simulink model "ArduCopter"  (R2016a)
settings: Solver=ode8  SolverMode=SingleTasking  StartTime=0.0  StopTime=endtime_selfdefine  FixedStep=0.0025  RelTol=1e-3
InitFcn:
  | %load QuadCopterParameters
values from neighbouring files (symbols this model uses):
  Discretetime_400Hz = 0.0025    [euler_roll_angle_cd.mat]
  flight_mode = 1    [flight_control_run.m]
undefined symbols (not defined in the file or in its folder): Cutoff_frequency_acc_z, D_acc_z, D_vel_x, D_vel_y, DEG_TO_RAD, Discretetime_1Hz, g, I_acc_z, I_vel_x, I_vel_y, Kp_angle, MotorLayout, P_acc_z, P_pos_x, P_pos_y, P_pos_z, P_vel_x, P_vel_y, P_vel_z, thrust_rpyt_down, thrust_rpyt_up
libraries: Lib_AC_AttitudeControl x26, Lib_AP_Math x26, Lib_AP_Motors x5, Lib_AC_PID x4, Lib_AP_AHRS x3, simulink x1
(part 2 of 2)

== system ArduCopter/loop/fast_loop/update_flight_mode/poshold_run/set_throttle_out/update_z_controller/pos_to_rate_z ==
  note: in cm，positive
  _ahrs : Inport
  _pos_target.z : Inport  Port=2
  Bus Selector : BusSelector  OutputSignals=NEDState.Position.zPos,NEDState.Velocity.zVel
  Gain : Gain  Gain=-100
  Gain2 : Gain  Gain=-100
  MATLAB Function1 : Lib_AC_AttitudeControl/MATLAB Function2
  Parameter1 : Constant  Value=P_pos_z  SampleTime=-1
  Parameter2 : Constant  Value=250  SampleTime=-1
  Scope : Scope  NumInputPorts=3
  Subtract : Sum  Inputs=+-
  rate_to_accel_z : Subsystem
  _throttle_in : Outport
  wires:
  _ahrs/1 -> rate_to_accel_z/3(_ahrs), Bus Selector/1
  Bus Selector/1 -> Gain/1  "<zPos>"
  _pos_target.z/1 -> Scope/1, Subtract/1
  Subtract/1 -> MATLAB Function1/1, Scope/3
  Parameter1/1 -> MATLAB Function1/2
  MATLAB Function1/1 -> rate_to_accel_z/1(_vel_target.z)
  Gain2/1 -> rate_to_accel_z/2(_vel_cur.z)
  Bus Selector/2 -> Gain2/1  "<zVel>"
  rate_to_accel_z/1(_throttle_in) -> _throttle_in/1
  Gain/1 -> Scope/2, Subtract/2
  Parameter2/1 -> MATLAB Function1/3

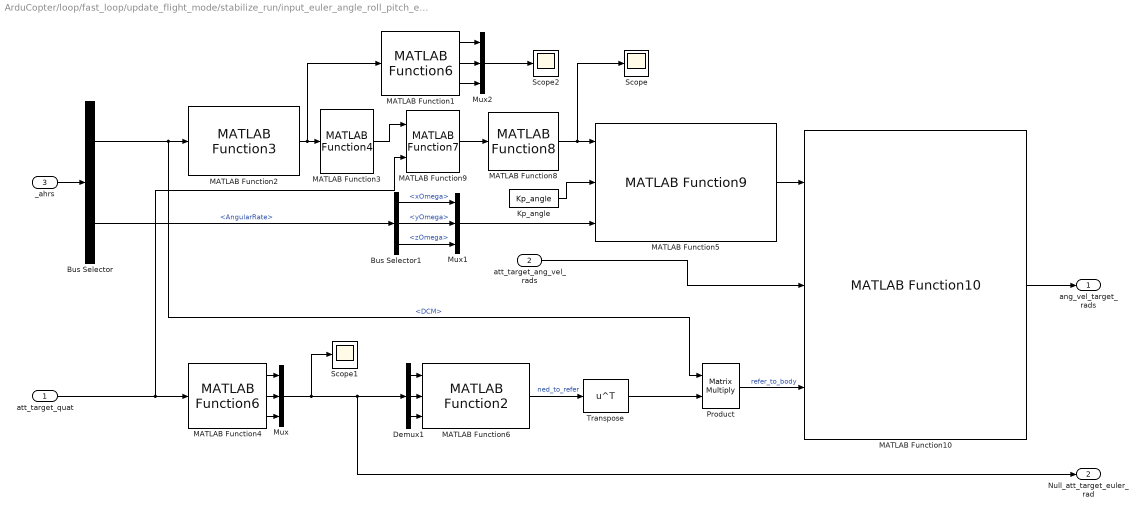
== system ArduCopter/loop/fast_loop/update_flight_mode/stabilize_run/input_euler_angle_roll_pitch_euler_rate_yaw_smooth/attitude_controller_run_euler/attitude_controller_run_quat ==
  att_target_quat : Inport
  att_target_ang_vel_rads : Inport  Port=2
  _ahrs : Inport  Port=3
  Bus Selector : BusSelector  OutputSignals=NEDState.Attitude.DCM,BodyState.AngularRate
  Bus Selector1 : BusSelector  OutputSignals=xOmega,yOmega,zOmega
  Demux1 : Demux  Outputs=3
  Kp_angle : Constant  Description=低通滤波器的时间常数  Value=Kp_angle
  MATLAB Function1 : Lib_AP_Math/MATLAB Function6
  MATLAB Function10 : Lib_AC_AttitudeControl/MATLAB Function10
  MATLAB Function2 : Lib_AP_Math/MATLAB Function3
  MATLAB Function3 : Lib_AP_Math/MATLAB Function4
  MATLAB Function4 : Lib_AP_Math/MATLAB Function6
  MATLAB Function5 : Lib_AC_AttitudeControl/MATLAB Function9
  MATLAB Function6 : Lib_AP_AHRS/MATLAB Function2
  MATLAB Function8 : Lib_AP_Math/MATLAB Function8
  MATLAB Function9 : Lib_AP_Math/MATLAB Function7
  Mux : Mux  Inputs=3
  Mux1 : Mux  Inputs=3
  Mux2 : Mux  Inputs=3
  Product : Product  Multiplication=Matrix(*)  RndMeth=Zero
  Scope : Scope
  Scope1 : Scope
  Scope2 : Scope
  Transpose : Math  Operator=transpose  SaturateOnIntegerOverflow=on
  ang_vel_target_rads : Outport
  Null_att_target_euler_rad : Outport  Port=2
  wires:
  Mux/1 -> Scope1/1, Null_att_target_euler_rad/1, Demux1/1
  MATLAB Function4/1 -> Mux/1
  MATLAB Function4/2 -> Mux/2
  MATLAB Function4/3 -> Mux/3
  MATLAB Function3/1 -> MATLAB Function9/1
  MATLAB Function10/1 -> ang_vel_target_rads/1
  att_target_ang_vel_rads/1 -> MATLAB Function10/2
  MATLAB Function5/1 -> MATLAB Function10/1
  MATLAB Function8/1 -> Scope/1, MATLAB Function5/1
  MATLAB Function9/1 -> MATLAB Function8/1
  MATLAB Function2/1 -> MATLAB Function1/1, MATLAB Function3/1
  att_target_quat/1 -> MATLAB Function9/2, MATLAB Function4/1
  Kp_angle/1 -> MATLAB Function5/2
  Bus Selector/1 -> Product/1, MATLAB Function2/1  "<DCM>"
  Demux1/1 -> MATLAB Function6/1
  Demux1/2 -> MATLAB Function6/2
  Demux1/3 -> MATLAB Function6/3
  MATLAB Function6/1 -> Transpose/1  "ned_to_refer"
  Transpose/1 -> Product/2
  Product/1 -> MATLAB Function10/3  "refer_to_body"
  _ahrs/1 -> Bus Selector/1
  Bus Selector/2 -> Bus Selector1/1  "<AngularRate>"
  Bus Selector1/2 -> Mux1/2  "<yOmega>"
  Bus Selector1/1 -> Mux1/1  "<xOmega>"
  Bus Selector1/3 -> Mux1/3  "<zOmega>"
  Mux1/1 -> MATLAB Function5/3
  MATLAB Function1/1 -> Mux2/1
  MATLAB Function1/2 -> Mux2/2
  MATLAB Function1/3 -> Mux2/3
  Mux2/1 -> Scope2/1

== system ArduCopter/loop/fast_loop/update_flight_mode/althold_run/set_throttle_out/update_z_controller/pos_to_rate_z/rate_to_accel_z ==
  _vel_target.z : Inport
  _vel_cur.z : Inport  Port=2
  _ahrs : Inport  Port=3
  Parameter1 : Constant  Value=P_vel_z  SampleTime=-1
  Product : Product
  Scope : Scope  NumInputPorts=3
  Subtract : Sum  Inputs=+-
  accel_to_throttle : Subsystem
  _throttle_in : Outport
  wires:
  _vel_target.z/1 -> Scope/1, Subtract/1
  _vel_cur.z/1 -> Subtract/2, Scope/2
  Subtract/1 -> Product/1, Scope/3
  Parameter1/1 -> Product/2
  Product/1 -> accel_to_throttle/1(_accel_target.z)  "_accel_target.z1"
  _ahrs/1 -> accel_to_throttle/2(_ahrs)
  accel_to_throttle/1(_throttle_in) -> _throttle_in/1

== system ArduCopter/loop/fast_loop/update_flight_mode/poshold_run/set_throttle_out/update_z_controller/pos_to_rate_z/rate_to_accel_z ==
  _vel_target.z : Inport
  _vel_cur.z : Inport  Port=2
  _ahrs : Inport  Port=3
  Parameter1 : Constant  Value=P_vel_z  SampleTime=-1
  Product : Product
  Scope : Scope  NumInputPorts=3
  Subtract : Sum  Inputs=+-
  accel_to_throttle : Subsystem
  _throttle_in : Outport
  wires:
  _vel_target.z/1 -> Scope/1, Subtract/1
  _vel_cur.z/1 -> Subtract/2, Scope/2
  Subtract/1 -> Product/1, Scope/3
  Parameter1/1 -> Product/2
  Product/1 -> accel_to_throttle/1(_accel_target.z)  "_accel_target.z1"
  _ahrs/1 -> accel_to_throttle/2(_ahrs)
  accel_to_throttle/1(_throttle_in) -> _throttle_in/1

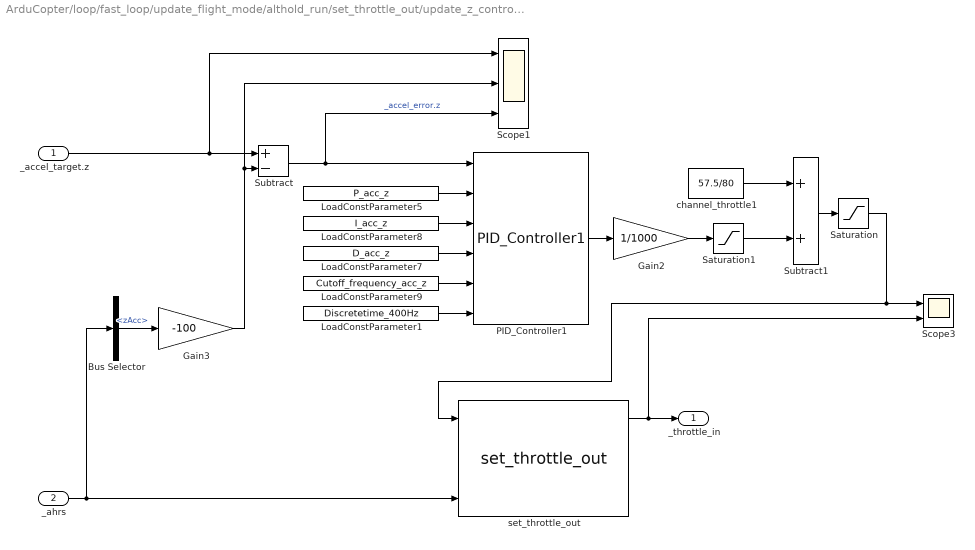
== system ArduCopter/loop/fast_loop/update_flight_mode/althold_run/set_throttle_out/update_z_controller/pos_to_rate_z/rate_to_accel_z/accel_to_throttle ==
  _accel_target.z : Inport
  _ahrs : Inport  Port=2
  Bus Selector : BusSelector  OutputSignals=NEDState.Acceleration.zAcc
  Gain2 : Gain  Gain=1/1000  SampleTime=0.0025
  Gain3 : Gain  Gain=-100  SampleTime=0.0025
  LoadConstParameter1 : Constant  Value=Discretetime_400Hz  SampleTime=-1
  LoadConstParameter5 : Constant  Value=P_acc_z  SampleTime=-1
  LoadConstParameter7 : Constant  Value=D_acc_z  SampleTime=-1
  LoadConstParameter8 : Constant  Value=I_acc_z  SampleTime=-1
  LoadConstParameter9 : Constant  Value=Cutoff_frequency_acc_z  SampleTime=-1
  PID_Controller1 : Lib_AC_PID/PID_Controller1  Description=PI控制器。
  Saturation : Saturate  UpperLimit=1  LowerLimit=0
  Saturation1 : Saturate  UpperLimit=1  LowerLimit=-57.5/80
  Scope1 : Scope  NumInputPorts=3
  Scope3 : Scope  NumInputPorts=2
  Subtract : Sum  Inputs=+-
  Subtract1 : Sum
  channel_throttle1 : Constant  Value=57.5/80  SampleTime=-1
  set_throttle_out : Lib_AC_AttitudeControl/set_throttle_out
  _throttle_in : Outport
  wires:
  Subtract/1 -> Scope1/3, PID_Controller1/1  "_accel_error.z"
  LoadConstParameter5/1 -> PID_Controller1/2
  LoadConstParameter8/1 -> PID_Controller1/3
  LoadConstParameter7/1 -> PID_Controller1/4
  LoadConstParameter9/1 -> PID_Controller1/5
  LoadConstParameter1/1 -> PID_Controller1/6
  PID_Controller1/1 -> Gain2/1
  channel_throttle1/1 -> Subtract1/1
  Subtract1/1 -> Saturation/1
  _ahrs/1 -> Bus Selector/1, set_throttle_out/3
  set_throttle_out/1 -> _throttle_in/1, Scope3/2
  Gain2/1 -> Saturation1/1
  Saturation/1 -> set_throttle_out/1, Scope3/1
  Bus Selector/1 -> Gain3/1  "<zAcc>"
  Gain3/1 -> Scope1/2, Subtract/2
  _accel_target.z/1 -> Scope1/1, Subtract/1
  Saturation1/1 -> Subtract1/2

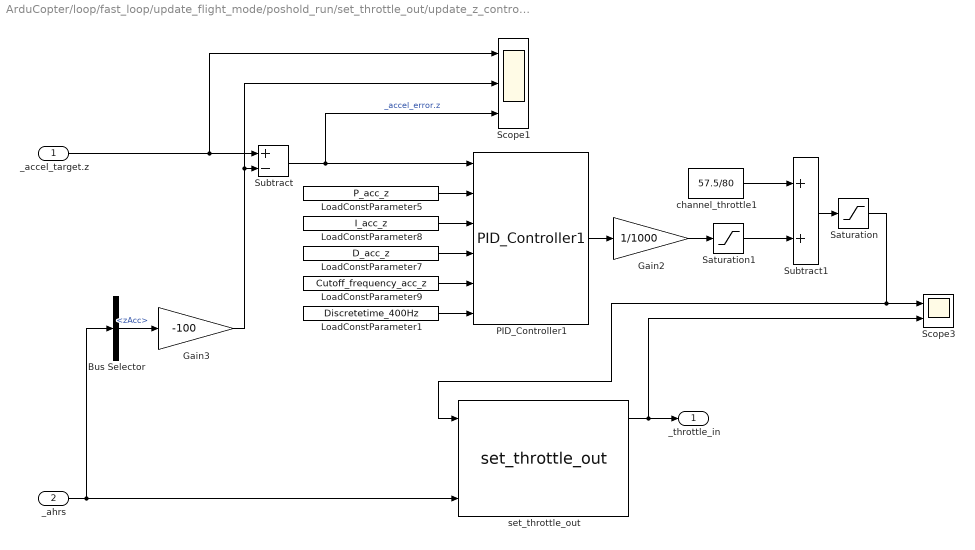
== system ArduCopter/loop/fast_loop/update_flight_mode/poshold_run/set_throttle_out/update_z_controller/pos_to_rate_z/rate_to_accel_z/accel_to_throttle ==
  _accel_target.z : Inport
  _ahrs : Inport  Port=2
  Bus Selector : BusSelector  OutputSignals=NEDState.Acceleration.zAcc
  Gain2 : Gain  Gain=1/1000  SampleTime=0.0025
  Gain3 : Gain  Gain=-100  SampleTime=0.0025
  LoadConstParameter1 : Constant  Value=Discretetime_400Hz  SampleTime=-1
  LoadConstParameter5 : Constant  Value=P_acc_z  SampleTime=-1
  LoadConstParameter7 : Constant  Value=D_acc_z  SampleTime=-1
  LoadConstParameter8 : Constant  Value=I_acc_z  SampleTime=-1
  LoadConstParameter9 : Constant  Value=Cutoff_frequency_acc_z  SampleTime=-1
  PID_Controller1 : Lib_AC_PID/PID_Controller1  Description=PI控制器。
  Saturation : Saturate  UpperLimit=1  LowerLimit=0
  Saturation1 : Saturate  UpperLimit=1  LowerLimit=-57.5/80
  Scope1 : Scope  NumInputPorts=3
  Scope3 : Scope  NumInputPorts=2
  Subtract : Sum  Inputs=+-
  Subtract1 : Sum
  channel_throttle1 : Constant  Value=57.5/80  SampleTime=-1
  set_throttle_out : Lib_AC_AttitudeControl/set_throttle_out
  _throttle_in : Outport
  wires:
  Subtract/1 -> Scope1/3, PID_Controller1/1  "_accel_error.z"
  LoadConstParameter5/1 -> PID_Controller1/2
  LoadConstParameter8/1 -> PID_Controller1/3
  LoadConstParameter7/1 -> PID_Controller1/4
  LoadConstParameter9/1 -> PID_Controller1/5
  LoadConstParameter1/1 -> PID_Controller1/6
  PID_Controller1/1 -> Gain2/1
  channel_throttle1/1 -> Subtract1/1
  Subtract1/1 -> Saturation/1
  _ahrs/1 -> Bus Selector/1, set_throttle_out/3
  set_throttle_out/1 -> _throttle_in/1, Scope3/2
  Gain2/1 -> Saturation1/1
  Saturation/1 -> set_throttle_out/1, Scope3/1
  Bus Selector/1 -> Gain3/1  "<zAcc>"
  Gain3/1 -> Scope1/2, Subtract/2
  _accel_target.z/1 -> Scope1/1, Subtract/1
  Saturation1/1 -> Subtract1/2

== matlab function ArduCopter/loop/LogData/datachange1 ==
  data: v3 input; q output
function q=datachange(v3)
q1=v3(1);
q2=v3(2);
q3=v3(3);
q=[q1;q2;q3];

== matlab function ArduCopter/loop/LogData/datachange3 ==
  data: v3 input; q output
function q=datachange(v3)
q1=v3(1);
q2=v3(2);
q3=v3(3);
q4=v3(4);
q5=v3(5);
q=[q1;q2;q3;q4;q5];

== matlab function ArduCopter/loop/LogData/datachange2 ==
  data: v3 input; q output
function q=datachange(v3)
q1=v3(1);
q2=v3(2);
q3=v3(3);
q4=v3(4);
q5=v3(5);
q=[q1;q2;q3;q4;q5];
